simulink library "Lib_VehDynMdls"  (R2016b)
settings: Solver=VariableStepAuto  StartTime=0.0  StopTime=10.0  RelTol=1e-3
undefined symbols (not defined in the file or in its folder): lf, lr
settings Model: Creator=sgopalswamy  LastModifiedBy=sgopalswamy

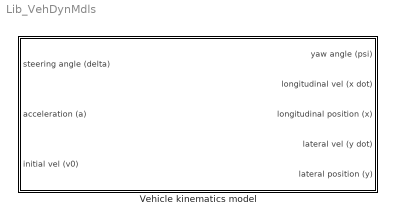
== system Lib_VehDynMdls ==
  Vehicle kinematics model : Subsystem

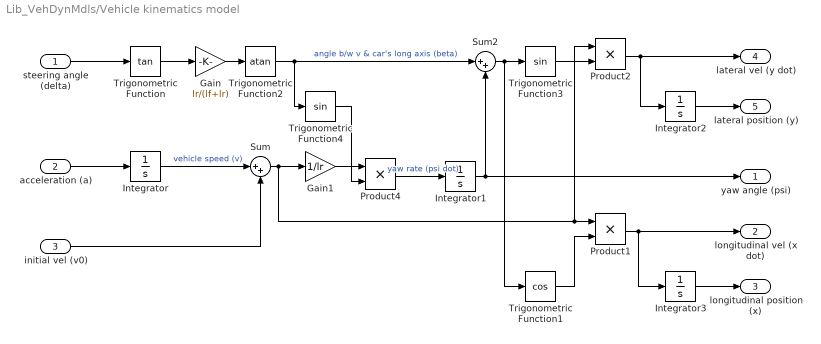
== system Lib_VehDynMdls/Vehicle kinematics model ==
  steering angle (delta) : Inport
  acceleration (a) : Inport  Port=2
  initial vel (v0) : Inport  Port=3
  Gain : Gain  Gain=lr/(lf+lr)
  Gain1 : Gain  Gain=1/lr
  Integrator{,1..3} (4 alike) : Integrator
  Product1 : Product
  Product2 : Product
  Product4 : Product
  Sum : Sum  Inputs=|++
  Sum2 : Sum  Inputs=|++
  Trigonometric Function : Trigonometry  Operator=tan
  Trigonometric Function1 : Trigonometry  Operator=cos
  Trigonometric Function2 : Trigonometry  Operator=atan
  Trigonometric Function3 : Trigonometry
  Trigonometric Function4 : Trigonometry
  yaw angle (psi) : Outport
  longitudinal vel (x dot) : Outport  Port=2
  longitudinal position (x) : Outport  Port=3
  lateral vel (y dot) : Outport  Port=4
  lateral position (y) : Outport  Port=5
  wires:
  acceleration (a)/1 -> Integrator/1
  steering angle (delta)/1 -> Trigonometric Function/1
  Trigonometric Function/1 -> Gain/1
  Gain/1 -> Trigonometric Function2/1
  Trigonometric Function2/1 -> Sum2/1, Trigonometric Function4/1  "angle b/w v & car's long axis (beta)"
  Gain1/1 -> Product4/1
  Product4/1 -> Integrator1/1  "yaw rate (psi dot)"
  Sum2/1 -> Trigonometric Function3/1, Trigonometric Function1/1
  Trigonometric Function1/1 -> Product1/2
  Product1/1 -> Integrator3/1, longitudinal vel (x dot)/1
  Trigonometric Function3/1 -> Product2/2
  Product2/1 -> Integrator2/1, lateral vel (y dot)/1
  Integrator2/1 -> lateral position (y)/1
  Integrator3/1 -> longitudinal position (x)/1
  Trigonometric Function4/1 -> Product4/2
  Integrator1/1 -> yaw angle (psi)/1, Sum2/2
  initial vel (v0)/1 -> Sum/2
  Sum/1 -> Product2/1, Product1/1, Gain1/1
  Integrator/1 -> Sum/1  "vehicle speed (v)"
